simulink model "n_metro_discret"  (Simulink 7.2)
settings: Solver=ode45  StartTime=0.0  StopTime=L  RelTol=1e-6
values from neighbouring files (symbols this model uses):
  Delta = 10    [lance_crash.m]
  K = (randn(N,1)*sigma_K)+Knom    [lance_crash.m]
  Ka = Kry(:,dim-1:dim:dim*N)    [lance_crash.m]
  Ki = Kry(:,1:dim:dim*N)*(dim-2)    [lance_crash.m]
  Kv = Kry(:,dim:dim:dim*N)    [lance_crash.m]
  L = 20    [lance_crash.m]
  M_ecart = 0    [lance_crash.m]
  N = 1    [lance_crash.m]
  Tau = (randn(N,1)*sigma_Tau)+Taunom    [lance_crash.m]
  Te = 1E-3    (= 0.001)    [lance_crash.m]
undefined symbols (not defined in the file or in its folder): DiscIntNeverNeededParam
settings Model: Creator=acco  LastModifiedBy=acco
settings DataIOCC: SignalLoggingName=sigsOut
settings DebuggingCC: SaveWithParameterizedLinksMsg=none  SignalResolutionControl=TryResolveAllWithWarning  SolverPrmCheckMsg=none  MultiTaskDSMMsg=warning  MultiTaskCondExecSysMsg=none  StrictBusMsg=None
settings HardwareCC: TargetUnknown=on
settings RTWCC: IncludeERTFirstTime=on

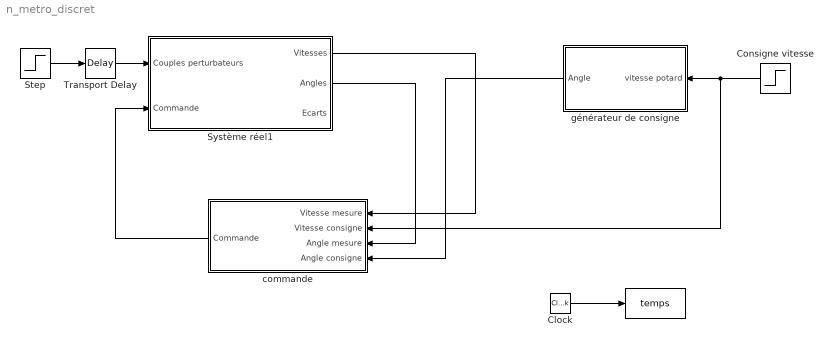
== system n_metro_discret ==
  " " : ToWorkspace  VariableName=temps  SampleTime=Te  SaveFormat=Array
  Clock : DigitalClock  SampleTime=Te
  Consigne vitesse : Step  Orientation=left  Time=L/2  Before=ones(N,1)*0  After=ones(N,1)  SampleTime=Te
  Step : Step  Time=L*0.1  Before=ones(N,1)*0  After=-ones(N,1)*0
  Système réel1 : Subsystem
  Transport Delay : TransportDelay  DelayTime=N-(1:N)
  commande : Subsystem  Orientation=left  TreatAsAtomicUnit=on
      settings: RTWSystemCode=Function  RTWFcnNameOpts=Use subsystem name  RTWFileNameOpts=Use subsystem name
  générateur de consigne : Subsystem  Orientation=left
  wires:
  Step/1 -> Transport Delay/1
  Consigne vitesse/1 -> commande/2(Vitesse consigne), générateur de consigne/1(vitesse potard)
  Système réel1/2(Angles) -> commande/3(Angle mesure)
  Clock/1 -> " "/1
  commande/1(Commande) -> Système réel1/2(Commande)
  Système réel1/1(Vitesses) -> commande/1(Vitesse mesure)
  générateur de consigne/1(Angle) -> commande/4(Angle consigne)
  Transport Delay/1 -> Système réel1/1(Couples perturbateurs)

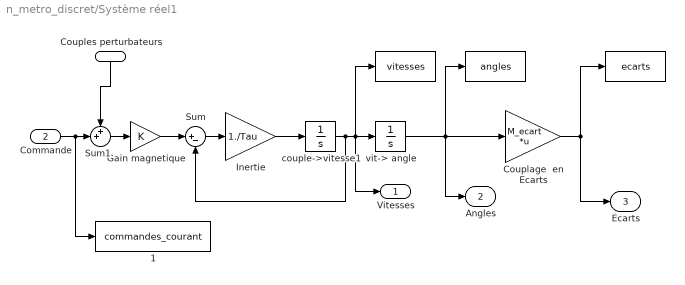
== system n_metro_discret/Système réel1 ==
  Couples perturbateurs : Inport  Orientation=down  OutDataType=sfix(16)  OutScaling=2^0
  Commande : Inport  Port=2  OutDataType=sfix(16)  OutScaling=2^0
  " " : ToWorkspace  VariableName=vitesses  SampleTime=Te  SaveFormat=Array
  "  " : ToWorkspace  VariableName=angles  SampleTime=Te  SaveFormat=Array
  "   " : ToWorkspace  VariableName=ecarts  SampleTime=Te  SaveFormat=Array
  "   1" : ToWorkspace  VariableName=commandes_courant  SampleTime=Te  SaveFormat=Array
  Couplage  en Ecarts : Gain  Gain=M_ecart  Multiplication=Matrix(K*u)  ParameterDataType=sfix(16)  ParameterScaling=2^0  OutDataType=sfix(16)  OutScaling=2^0  SaturateOnIntegerOverflow=on  OutDataTypeStr=Inherit: Same as input  ParamDataTypeStr=Inherit: Same as input
  Gain magnetique : Gain  Gain=K  ParameterDataType=sfix(16)  ParameterScaling=2^0  OutDataType=sfix(16)  OutScaling=2^0  SaturateOnIntegerOverflow=on  OutDataTypeStr=Inherit: Same as input  ParamDataTypeStr=Inherit: Same as input
  Inertie : Gain  Gain=1./Tau  ParameterDataType=sfix(16)  ParameterScaling=2^0  OutDataType=sfix(16)  OutScaling=2^0  SaturateOnIntegerOverflow=on  OutDataTypeStr=Inherit: Same as input  ParamDataTypeStr=Inherit: Same as input
  Sum : Sum  Inputs=|+-  OutDataType=sfix(16)  OutScaling=2^0  SaturateOnIntegerOverflow=on
  Sum1 : Sum  Inputs=++|  OutDataType=sfix(16)  OutScaling=2^0  SaturateOnIntegerOverflow=on
  couple->vitesse1 : Integrator  InitialCondition=zeros(N,1)
  vit-> angle : Integrator  InitialCondition=(0:N-1)*Delta
  Vitesses : Outport  OutDataType=sfix(16)  OutScaling=2^0
  Angles : Outport  Port=2  OutDataType=sfix(16)  OutScaling=2^0
  Ecarts : Outport  Port=3  OutDataType=sfix(16)  OutScaling=2^0
  wires:
  vit-> angle/1 -> "  "/1, Angles/1, Couplage  en Ecarts/1
  Commande/1 -> "   1"/1, Sum1/2
  Couplage  en Ecarts/1 -> "   "/1, Ecarts/1
  Inertie/1 -> couple->vitesse1/1
  Gain magnetique/1 -> Sum/1
  Sum/1 -> Inertie/1
  couple->vitesse1/1 -> vit-> angle/1, Vitesses/1, " "/1, Sum/2
  Sum1/1 -> Gain magnetique/1
  Couples perturbateurs/1 -> Sum1/1

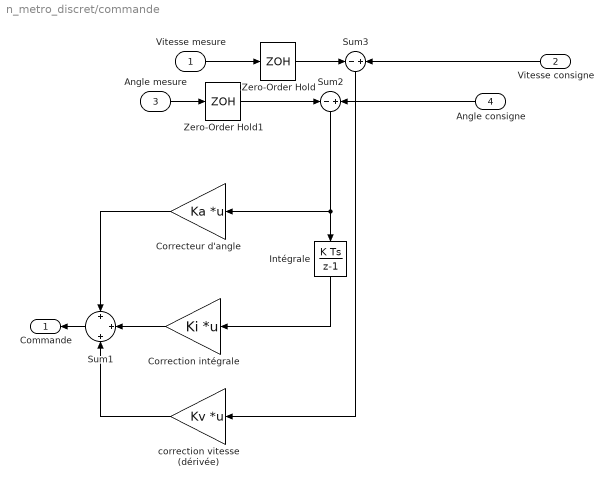
== system n_metro_discret/commande ==
  Vitesse mesure : Inport  OutDataType=sfix(16)  OutScaling=2^0
  Vitesse consigne : Inport  Orientation=left  Port=2  OutDataType=sfix(16)  OutScaling=2^0
  Angle mesure : Inport  Port=3  OutDataType=sfix(16)  OutScaling=2^0
  Angle consigne : Inport  Orientation=left  Port=4  OutDataType=sfix(16)  OutScaling=2^0
  Correcteur d'angle : Gain  Orientation=left  Gain=Ka  Multiplication=Matrix(K*u)  ParameterDataType=sfix(16)  ParameterScaling=2^0  OutDataType=sfix(16)  OutScaling=2^0  SaturateOnIntegerOverflow=on  OutDataTypeStr=Inherit: Same as input  ParamDataTypeStr=Inherit: Same as input
  Correction intégrale : Gain  Orientation=left  Gain=Ki  Multiplication=Matrix(K*u)  ParameterDataType=sfix(16)  ParameterScaling=2^0  OutDataType=sfix(16)  OutScaling=2^0  SaturateOnIntegerOverflow=on  OutDataTypeStr=Inherit: Same as input  ParamDataTypeStr=Inherit: Same as input
  Intégrale : DiscreteIntegrator  Orientation=down  InitialCondition=zeros(N,1)  SampleTime=Te  ICPrevOutput=DiscIntNeverNeededParam  ICPrevScaledInput=DiscIntNeverNeededParam
  Sum1 : Sum  Orientation=left  Inputs=+|+|+  OutDataType=sfix(16)  OutScaling=2^0  SaturateOnIntegerOverflow=on
  Sum2 : Sum  Orientation=down  Inputs=-|+  OutDataType=sfix(16)  OutScaling=2^0  SaturateOnIntegerOverflow=on
  Sum3 : Sum  Orientation=down  Inputs=-|+  OutDataType=sfix(16)  OutScaling=2^0  SaturateOnIntegerOverflow=on
  Zero-Order Hold : ZeroOrderHold  SampleTime=Te
  Zero-Order Hold1 : ZeroOrderHold  SampleTime=Te
  correction vitesse (dérivée) : Gain  Orientation=left  Gain=Kv  Multiplication=Matrix(K*u)  ParameterDataType=sfix(16)  ParameterScaling=2^0  OutDataType=sfix(16)  OutScaling=2^0  SaturateOnIntegerOverflow=on  OutDataTypeStr=Inherit: Same as input  ParamDataTypeStr=Inherit: Same as input
  Commande : Outport  Orientation=left
  wires:
  Sum2/1 -> Intégrale/1, Correcteur d'angle/1
  Correcteur d'angle/1 -> Sum1/1
  Sum3/1 -> correction vitesse (dérivée)/1
  Intégrale/1 -> Correction intégrale/1
  correction vitesse (dérivée)/1 -> Sum1/3
  Correction intégrale/1 -> Sum1/2
  Vitesse consigne/1 -> Sum3/2
  Angle consigne/1 -> Sum2/2
  Vitesse mesure/1 -> Zero-Order Hold/1
  Angle mesure/1 -> Zero-Order Hold1/1
  Sum1/1 -> Commande/1
  Zero-Order Hold/1 -> Sum3/1
  Zero-Order Hold1/1 -> Sum2/1

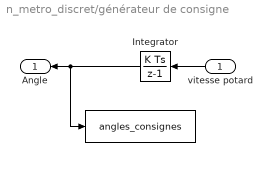
== system n_metro_discret/générateur de consigne ==
  vitesse potard : Inport  Orientation=left  OutDataType=sfix(16)  OutScaling=2^0
  "  " : ToWorkspace  VariableName=angles_consignes  SampleTime=Te  SaveFormat=Array
  Integrator : DiscreteIntegrator  Orientation=left  InitialCondition=[0:N-1]'*Delta  SampleTime=Te  ICPrevOutput=DiscIntNeverNeededParam  ICPrevScaledInput=DiscIntNeverNeededParam
  Angle : Outport  Orientation=left
  wires:
  Integrator/1 -> "  "/1, Angle/1
  vitesse potard/1 -> Integrator/1
